simulink model "test_udp"  (R2013b)
settings: Solver=ode3  StartTime=0.0  StopTime=inf  FixedStep=0.01  RelTol=1e-3
InitFcn:
  | echoudp('off')
  | 
  | remote_host = '192.168.1.110';
  | remote_port = 9701
  | echoudp('on', remote_port)
  | local_port_tx = 9801:9899;
  | local_port_rx = 9801:9899;
  | 
  | 
  | if license('checkout','instrument_control_toolbox')
  |   disp('license available')
  | else
  |   disp('no license available')
  | end
  | 
  | Fscale = 0.25
libraries: TEsim_utils x6
settings Model: Creator=rnc4  LastModifiedBy=rnc4

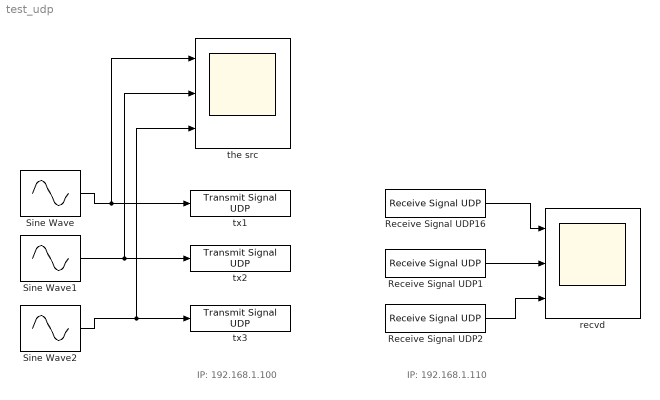
== system test_udp ==
  note: IP: 192.168.1.100
  note: IP: 192.168.1.110
  Receive Signal UDP1 : TEsim_utils/Communications/Receive Signal UDP  Host=localhost  Port=remote_port  LocalPort=local_port_rx(2)  SampleTime=0.01
  Receive Signal UDP16 : TEsim_utils/Communications/Receive Signal UDP  Host=localhost  Port=remote_port  LocalPort=local_port_rx(1)  SampleTime=0.01
  Receive Signal UDP2 : TEsim_utils/Communications/Receive Signal UDP  Host=localhost  Port=remote_port  LocalPort=local_port_rx(3)  SampleTime=0.01
  Sine Wave : Sin  Frequency=Fscale*2*pi  SampleTime=0
  Sine Wave1 : Sin  Frequency=Fscale*4*pi  Phase=30  SampleTime=0
  Sine Wave2 : Sin  Frequency=Fscale*6*pi  Phase=60  SampleTime=0
  recvd : Scope  NumInputPorts=3
      settings: TimeRange=10  YMin=-1~-1~-1  YMax=1~1~1
  the src : Scope  NumInputPorts=3
      settings: YMin=-5~-5~-5  YMax=5~5~5
  tx1 : TEsim_utils/Communications/Transmit Signal UDP  Priority=100  Ts=0.01  Host=localhost  Port=remote_port  LocalPort=local_port_tx(1)  EnableBlockingMode=off
  tx2 : TEsim_utils/Communications/Transmit Signal UDP  Priority=100  Ts=0.01  Host=localhost  Port=remote_port  LocalPort=local_port_tx(2)  EnableBlockingMode=off
  tx3 : TEsim_utils/Communications/Transmit Signal UDP  Priority=100  Ts=0.01  Host=localhost  Port=remote_port  LocalPort=local_port_tx(3)  EnableBlockingMode=off
  wires:
  Receive Signal UDP16/1 -> recvd/1
  Receive Signal UDP1/1 -> recvd/2
  Receive Signal UDP2/1 -> recvd/3
  Sine Wave/1 -> the src/1, tx1/1
  Sine Wave1/1 -> tx2/1, the src/2
  Sine Wave2/1 -> tx3/1, the src/3
